simulink model "Model"  (R2021a)
settings: Solver=ode4  StartTime=0.0  StopTime=inf  FixedStep=Ts  RelTol=1e-3
PreLoadFcn:
  | filepath  = fileparts(get_param(bdroot, 'FileName'))
  | cd(filepath);
values from neighbouring files (symbols this model uses):
  A_GRotation = [0 0 0]    [Parameter_PX4.m]
  ACC_UserFault = 0    [Parameter_PX4.m]
  ACCDrift = 0.0    (= 0)    [Parameter_PX4.m]
  ACCNoise = 1.0    (= 1)    [Parameter_PX4.m]
  accnoisegain = 0    [Parameter_PX4.m]
  ACCScale = 1.0    (= 1)    [Parameter_PX4.m]
  BaroNoise = 1.0    (= 1)    [Parameter_PX4.m]
  GyroDrift = 0.0    (= 0)    [Parameter_PX4.m]
  GyroNoise = 1.0    (= 1)    [Parameter_PX4.m]
  GyroScale = 1.0    (= 1)    [Parameter_PX4.m]
  MagDrift = 0.0    (= 0)    [Parameter_PX4.m]
  MagNoise = 1.0    (= 1)    [Parameter_PX4.m]
  MagRotation = [0 0 0]    [Parameter_PX4.m]
  MagScale = 1.0    (= 1)    [Parameter_PX4.m]
  ModelInit_GroundSlope = [0,0]    [Parameter_PX4.m]
  ModelInit_RPM = 0    [Parameter_PX4.m]
  ModelParam_envAltitude = -100    [Parameter_PX4.m]
  ModelParam_GlobalNoiseGainSwitch = 0.4    [Parameter_PX4.m]
  ModelParam_GPSEphFinal = 0.3    [Parameter_PX4.m]
  ModelParam_GPSEpvFinal = 0.4    [Parameter_PX4.m]
  ModelParam_GPSFix3DFix = 3    [Parameter_PX4.m]
  ModelParam_GPSSatsVisible = 10    [Parameter_PX4.m]
  ModelParam_motorCr = 842.1    [Parameter_PX4.m]
  ModelParam_motorJm = 0.0001287    [Parameter_PX4.m]
  ModelParam_motorMinThr = 0.05    [Parameter_PX4.m]
  ModelParam_motorT = 0.0214    [Parameter_PX4.m]
  ModelParam_motorWb = 22.83    [Parameter_PX4.m]
  ModelParam_noiseBaroCoupleWithSpeed = 0    [Parameter_PX4.m]
  ModelParam_noiseUpperWindBodyRatio = 0    [Parameter_PX4.m]
  ModelParam_rotorCm = 2.783e-07    [Parameter_PX4.m]
  ModelParam_rotorCt = 1.681e-05    [Parameter_PX4.m]
  ModelParam_uavCCm = [0.0035 0.0039 0.0034]    [Parameter_PX4.m]
  ModelParam_uavCd = 0.055    [Parameter_PX4.m]
  ModelParam_uavDearo = 0.12    [Parameter_PX4.m]
  ModelParam_uavMass = 1.515    [Parameter_PX4.m]
  ModelParam_uavR = 0.225    [Parameter_PX4.m]
  ModelParam_uavType = int8(3)    [Parameter_PX4.m]
  MyNoiseGain = [2.5;3;4].*3    [Parameter_PX4.m]
  PWMNoiseGain = [10;15;3]    [Parameter_PX4.m]
  TemperatureConstant = 25.0    (= 25)    [Parameter_PX4.m]
  Ts = 1/2000    (= 0.0005)    [Parameter_PX4.m]
  TypeMotorAngMatrix = [     [pi/3 pi -pi/3 0 0 0 0 0];     [pi/3 pi -pi/3 0 0 0 0 0];     [pi/4 pi/4+pi pi/4+3*pi/2 pi/4+pi/2 0 0 0 0];     [pi/2 3*pi/2 0 pi 0 0 0 0];     [pi/2 3/2*pi 3/2*pi+pi/3 pi/2+pi/3 pi/2-pi/3 3/2*pi-pi/3 0 0];     [0 pi pi+pi/3 pi/3 -pi/3 pi-pi/3 0 0];     [pi/3 pi/3 pi pi -pi/3 -pi/3 0 0];     [pi/8 pi+pi/8 pi/8+pi/4 pi-pi/8 -pi/8 3/2*pi-pi/8 3/2*pi+pi/8 pi/2+pi/8];     [0 pi pi/4 3/4*pi -pi/4 ...(+86 chars)    [Parameter_PX4.m]
  TypeMotorDirMatrix = [     [-1 -1 -1 0 0 0 0 0];     [1 1 1 0 0 0 0 0];     [-1 -1 1 1 0 0 0 0];     [-1 -1 1 1 0 0 0 0];     [1 -1 1 -1 -1 1 0 0];     [1 -1 1 -1 -1 1 0 0];     [1 -1 1 -1 1 -1 0 0];     [1 1 -1 -1 -1 -1 1 1];     [1 1 -1 -1 -1 -1 1 1];     [-1 1 -1 1 -1 1 -1 1]; ]'    [Parameter_PX4.m]
  TypeMotorNonVector = int8([3;3;4;4;6;6;6;8;8;8])    [Parameter_PX4.m]
undefined symbols (not defined in the file or in its folder): Earth, ModelParam_GPSEpvInitial, ModelParam_GPSEpvTimeConstant, ModelParam_noiseGPSSampTime, ModelParam_noisePowerIMU, ModelParam_noisePowerOffGainAccel, ModelParam_noisePowerOffGainAccelZ, ModelParam_noisePowerOffGainGyro, ModelParam_noisePowerOffGainGyroZ, ModelParam_noisePowerOffGainMag, ModelParam_noisePowerOffGainMagZ, ModelParam_noisePowerOnGainAccel, ModelParam_noisePowerOnGainAccelZ, ModelParam_noisePowerOnGainGyro, ModelParam_noisePowerOnGainGyroZ, ModelParam_noisePowerOnGainMag, ModelParam_noisePowerOnGainMagZ, ModelParam_noiseUpperGPS, ModelParam_timeSamp, Newton, Raphson, WGS84
libraries: simulink x11, sharedtransform x7, aerolibutil x4, aerolibtransform2 x4, aerolibasang x3, simulink_extras x2, etargetslib x2, aerolibatmos2 x2, shared6dof x1, aerolibconvert2 x1, aerolibobsolete x1, aerolibnav x1
(part 3 of 3)

== matlab function Model/6DOF/CaliModel/Ground Model ==
  settings: updateMethod=DISCRETE
  data: wb input; F1 output; M1 output; Quet input; isRot input; rotSpeed input; rotTime input; step input; clock input
function [F1,M1] = fcn(wb,Quet,isRot,rotSpeed,rotTime,step,clock)
% This is a ground model that can provides reaction force and reaction torque

%静态变量，作为一个计数器，记录进入当前step后的执行周期
persistent lastClock;
if isempty(lastClock)
    lastClock=0;
end

%静态变量，作为一个标志位，记录上次step步骤
persistent lastStep;
if isempty(lastStep)
    lastStep=uint8(1);
end

% 如果仿真步骤改变，则重新技术
if lastStep~=step
    lastClock=clock;
end

% 进入当前step的时间
t = clock-lastClock;


F1=[0;0;0];
M1=[0;0;0];

if isRot<0.5 %期望角度模式，则直接反馈
    M1=-5*[Quet(2);Quet(3);Quet(4)]-1*wb;  

else %期望旋转模式
    if t<rotTime
        M1=0.2*(rotSpeed-wb);  
    else
        M1=-5*[Quet(2);Quet(3);Quet(4)]-1*wb;  
    end
end


lastStep=step;

== matlab function Model/6DOF/CaliModel/MATLAB Function ==
  data: step input; desiredEuler output; Accel_Mag input; isRot output; rotSpeed output; rotTime output
function [desiredEuler,isRot,rotSpeed,rotTime] = fcn(step, Accel_Mag)

isRot=0; % 是否进入旋转模式（适用于磁力计）
rotTime=0; % 旋转的时间
rotSpeed=[0,0,0]; % 旋转的角速度

if Accel_Mag ==0 %加速度计校正模式
    switch step
        %% 加速度计
        case 1 %level 让飞机回到水平位置
            desiredEuler=[0,0,8.88*pi/180];

        case 2 %left side roll=-90 % 向左滚动到90度位置

            desiredEuler=[pi/2,0,0];

        case 3 %right side roll=90

            desiredEuler=[-pi/2,0,0];

        case 4 % 回到水平位置
            desiredEuler=[0,0,0];

        case 5 %nose down pitch=-90 头朝下
            
            desiredEuler=[0,-pi/2,0];

        case 6 %nose up pitch=90 头朝上

            desiredEuler=[0,pi/2,0];

       case 7 %level 回到水平
            desiredEuler=[0,0,0];
            
       case 8 %back side 底朝天
            desiredEuler=[pi,0,0];
%             desiredEuler=[0,pi,0];

        otherwise % 默认水平
            desiredEuler=[0,0,0];
    end
else
    switch step
        %% 向上阶段
        case 1 %up
            desiredEuler=[0,0,0];
        case 2 %up          
            %最终期望角度
            desiredEuler=[0,0,0];
            isRot=1; %进入旋转模式
            rotSpeed=[0,0,0.5]; % z轴方向转，0.5弧度每秒
            %旋转2pi度
            rotTime=6*pi/0.5; % 旋转时间，超过这个时间后会自动归位到desiredEuler
         case 3 %
            desiredEuler=[0,0,0];

        %% 向后
         case 4 %
            % 机身调整到朝后
            desiredEuler=[0,pi/2,0];
         case 5 %
            %最终期望角度
            desiredEuler=[0,pi/2,0];
            isRot=1; %进入旋转模式
            rotSpeed=[0.5,0,0]; % z轴方向转，0.5弧度每秒
            %旋转2*pi度
            rotTime=2*pi/0.5; % 旋转时间，超过这个时间后会自动归位到desiredEuler
         case 6 %
            desiredEuler=[0,pi/2,0];

         %% 向前
         case 7
            %机身调整到朝前
            desiredEuler=[0,-pi/2,0];
         case 8
            %最终期望角度
            desiredEuler=[0,-pi/2,0];
            isRot=1; %进入旋转模式
            rotSpeed=[0.5,0,0]; % z轴方向转，0.5弧度每秒
            %旋转2*pi度
            rotTime=2*pi/0.5; % 旋转时间，超过这个时间后会自动归位到desiredEuler
         case 9
            desiredEuler=[0,-pi/2,0];
            
        %% 向右
        case 10
             %机身调整到朝右
            desiredEuler=[pi/2,0,0];
        case 11
            %最终期望角度
            desiredEuler=[pi/2,0,0];
            isRot=1; %进入旋转模式
            rotSpeed=[0,0.5,0]; % z轴方向转，0.5弧度每秒
            %旋转2*pi度
            rotTime=2*pi/0.5; % 旋转时间，超过这个时间后会自动归位到desiredEuler
        case 12
            desiredEuler=[pi/2,0,0];

        %% 向左
        case 13
             %机身调整到朝左
            desiredEuler=[-pi/2,0,0];
        case 14
            %最终期望角度
            desiredEuler=[-pi/2,0,0];
            isRot=1; %进入旋转模式
            rotSpeed=[0,0.5,0]; % z轴方向转，0.5弧度每秒
            %旋转2*pi度
            rotTime=2*pi/0.5; % 旋转时间，超过这个时间后会自动归位到desiredEuler
        case 15
             desiredEuler=[-pi/2,0,0];
             
        %% 向下
        case 16
            %机身调整到朝下
            desiredEuler=[pi,0,0];
        case 17
            %最终期望角度
            desiredEuler=[pi,0,0];
            isRot=1; %进入旋转模式
            rotSpeed=[0,0,0.5]; % z轴方向转，0.5弧度每秒
            %旋转2*pi度
            rotTime=2*pi/0.5; % 旋转时间，超过这个时间后会自动归位到desiredEuler
        case 18
            desiredEuler=[pi,0,0];
         
        %% 
        otherwise
            desiredEuler=[0,0,0];
    end
end

== matlab function Model/SensorModel1/HILSensorMavModel1/MATLAB Function1 ==
  settings: updateMethod=DISCRETE
  data: timestamp input; noisegain input; y output; isact input; MyNoiseGain input
function y = fcn(timestamp, noisegain, isact, MyNoiseGain)

persistent last_time;
persistent count;

if isempty(count)
    count = 1;
end

if isempty(last_time)
    last_time = uint32(0);
end

if isact == 1.0
    if timestamp - last_time >= 20000  %10000 
        count = count + 1;       
        if count >= 2264
            count = 2264;
        end
        last_time = timestamp;       
    end
    s = [noisegain(count)*MyNoiseGain(1) noisegain(count)*MyNoiseGain(2) noisegain(count)*MyNoiseGain(3)];
else
    count = 0;
    s = [1 1 1];
end

y = s;

== matlab function Model/SensorModel1/HILSensorMavModel1/MATLAB Function ==
  data: temp input; Ab input; y output
function y = fcn(temp,Ab)

fitx = [-0.000000449538784   0.000050093027511  -0.005778015129211  -0.030104356819423];
fity = [0.000001962846074  -0.000193070271193   0.002231956222873   0.121722371351393 ];
fitz = [0.000005986700621  -0.000654115347298   0.024844214728420  -0.529514740245635 ];

accx = Ab(1) + fitx(1)*temp^3 + fitx(2)*temp^2 + fitx(3)*temp + fitx(4);
accy = Ab(2) + fity(1)*temp^3 + fity(2)*temp^2 + fity(3)*temp + fity(4);
accz = Ab(3) + fitz(1)*temp^3 + fitz(2)*temp^2 + fitz(3)*temp + fitz(4);

y = [accx accy accz];

== matlab function Model/SensorModel1/HILSensorMavModel1/AccelNoiseGainFunction1 ==
  data: theta input; Gain output; gain input
function Gain = fcn(theta,gain)
%#codegen
if theta>0.1
    Gain = [gain(1)*theta;gain(2)*theta;gain(3)*theta];
else
    Gain = [1;1;1];
end

== matlab function Model/SensorModel1/HILGPSModel/GenCogVel ==
  data: v output; u input; cot output
function [v,cot] = Ang360(u)
v=norm(u(1:2));

if v < 1
    cot = 0;
else
    cot=atan2d(u(2),u(1));
end
 
if cot<0
    cot=cot+360;
end

== matlab function Model/SensorModel1/HILGPSModel/MATLAB Function ==
  data: eph input; FixType output
function FixType = fcn(eph)
if eph <= 2
    FixType=3;
elseif eph <= 4
    FixType=2;
else
    FixType=0;
end

== matlab function Model/SensorModel1/HILSensorMavModel1/AccelNoiseGainFunction ==
  data: theta input; Gain output; ModelParam_noisePowerOnGainAccel parameter; ModelParam_noisePowerOffGainAccel parameter; ModelParam_noisePowerOnGainAccelZ parameter; ModelParam_noisePowerOffGainAccelZ parameter
function Gain = fcn(theta, ModelParam_noisePowerOnGainAccel, ModelParam_noisePowerOffGainAccel,ModelParam_noisePowerOnGainAccelZ, ModelParam_noisePowerOffGainAccelZ)
%#codegen
if theta>0.1
Gain = [ModelParam_noisePowerOnGainAccel;ModelParam_noisePowerOnGainAccel;ModelParam_noisePowerOnGainAccelZ];
else
    Gain = [ModelParam_noisePowerOffGainAccel;ModelParam_noisePowerOffGainAccel;ModelParam_noisePowerOffGainAccelZ];
end

== matlab function Model/SensorModel1/HILSensorMavModel1/GyroNoiseGainFunction ==
  data: theta input; Gain output; ModelParam_noisePowerOnGainGyro parameter; ModelParam_noisePowerOffGainGyro parameter; ModelParam_noisePowerOnGainGyroZ parameter; ModelParam_noisePowerOffGainGyroZ parameter
function Gain = fcn(theta, ModelParam_noisePowerOnGainGyro, ModelParam_noisePowerOffGainGyro, ModelParam_noisePowerOnGainGyroZ, ModelParam_noisePowerOffGainGyroZ)
%#codegen
if theta>0.1
    Gain = [ModelParam_noisePowerOnGainGyro;ModelParam_noisePowerOnGainGyro;ModelParam_noisePowerOnGainGyroZ];
else
    Gain = [ModelParam_noisePowerOffGainGyro;ModelParam_noisePowerOffGainGyro;ModelParam_noisePowerOffGainGyroZ];
end

== matlab function Model/SensorModel1/HILSensorMavModel1/MagNoiseGainFunction ==
  data: theta input; Gain output; ModelParam_noisePowerOnGainMag parameter; ModelParam_noisePowerOffGainMag parameter; ModelParam_noisePowerOnGainMagZ parameter; ModelParam_noisePowerOffGainMagZ parameter
function Gain = fcn(theta, ModelParam_noisePowerOnGainMag, ModelParam_noisePowerOffGainMag, ModelParam_noisePowerOnGainMagZ, ModelParam_noisePowerOffGainMagZ)
%#codegen
if theta>0.1
    Gain = [ModelParam_noisePowerOnGainMag;ModelParam_noisePowerOnGainMag;ModelParam_noisePowerOnGainMagZ];
else
    Gain = [ModelParam_noisePowerOffGainMag;ModelParam_noisePowerOffGainMag;ModelParam_noisePowerOffGainMagZ];
end
